simulink model "PICtrl"  (R2020b)
settings: Solver=VariableStepAuto  StartTime=0.0  StopTime=50  RelTol=1e-3
model workspace (MAT data in the model file):
  Ki = 36
  Kp = 25
undefined symbols (not defined in the file): ki, Ts
settings Model: Creator=ADMIN  LastModifiedBy=ADMIN

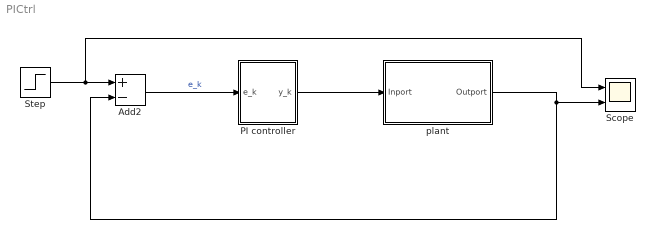
== system PICtrl ==
  Add2 : Sum  Inputs=+-
  PI controller : Subsystem  TreatAsAtomicUnit=on
  Scope : Scope  NumInputPorts=2
  Step : Step  Time=0  After=5  SampleTime=0
  plant : Subsystem  TreatAsAtomicUnit=on
  wires:
  Step/1 -> Scope/1, Add2/1
  plant/1(Outport) -> Add2/2, Scope/2
  Add2/1 -> PI controller/1(e_k)  "e_k"
  PI controller/1(y_k) -> plant/1(Inport)

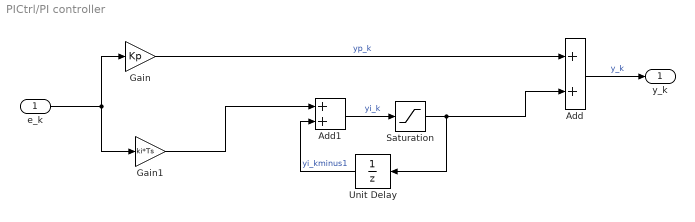
== system PICtrl/PI controller ==
  e_k : Inport
  Add : Sum
  Add1 : Sum
  Gain : Gain  Gain=Kp
  Gain1 : Gain  Gain=ki*Ts
  Saturation : Saturate  UpperLimit=1  LowerLimit=-1
  Unit Delay : UnitDelay  SampleTime=-1  HasFrameUpgradeWarning=on
  y_k : Outport
  wires:
  e_k/1 -> Gain1/1, Gain/1
  Gain1/1 -> Add1/1
  Gain/1 -> Add/1  "yp_k"
  Unit Delay/1 -> Add1/2  "yi_kminus1"
  Add/1 -> y_k/1  "y_k"
  Saturation/1 -> Unit Delay/1, Add/2
  Add1/1 -> Saturation/1  "yi_k"

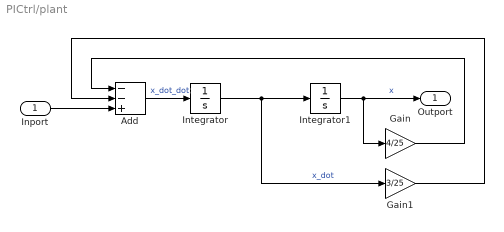
== system PICtrl/plant ==
  Inport : Inport
  Add : Sum  Inputs=--+
  Gain : Gain  Gain=4/25
  Gain1 : Gain  Gain=3/25
  Integrator : Integrator
  Integrator1 : Integrator
  Outport : Outport
  wires:
  Inport/1 -> Add/3
  Integrator/1 -> Gain1/1, Integrator1/1  "x_dot"
  Add/1 -> Integrator/1  "x_dot_dot"
  Integrator1/1 -> Outport/1, Gain/1  "x"
  Gain/1 -> Add/1
  Gain1/1 -> Add/2
